simulink model "model2017b"  (R2017b)
settings: Solver=VariableStepAuto  StartTime=0.0  StopTime=10.0  MaxStep=0.001  RelTol=1e-3
values from neighbouring files (symbols this model uses):
  F = 0    [main.m]
  g = 9.81    [main.m]
  l = 1    [main.m]
  M = 0.5    [main.m]
  m = 0.5    [main.m]
  T = 0    [main.m]
settings Model: Creator=mc764  LastModifiedBy=mc764

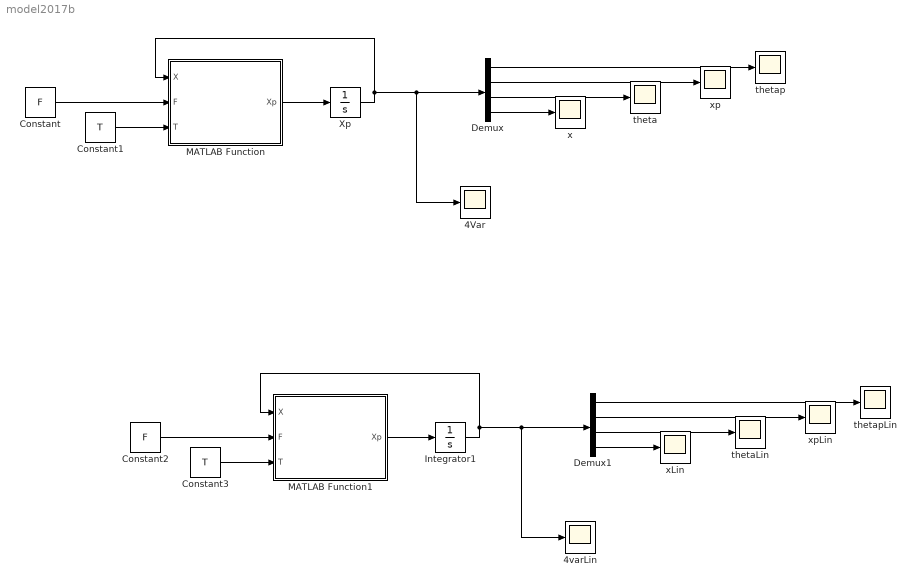
== system model2017b ==
  4Var : Scope
  4varLin : Scope
  Constant : Constant  Value=F
  Constant1 : Constant  Value=T
  Constant2 : Constant  Value=F
  Constant3 : Constant  Value=T
  Demux : Demux
  Demux1 : Demux
  Integrator1 : Integrator  InitialCondition=[0 0 180 0]
  MATLAB Function : MATLAB Function  TreatAsAtomicUnit=on
  MATLAB Function1 : MATLAB Function  TreatAsAtomicUnit=on
  Xp : Integrator  InitialCondition=[0 0 180 0]
  theta : Scope
  thetaLin : Scope
  thetap : Scope
  thetapLin : Scope
  x : Scope
  xLin : Scope
  xp : Scope
  xpLin : Scope
  wires:
  MATLAB Function/1(Xp) -> Xp/1
  Xp/1 -> 4Var/1, Demux/1, MATLAB Function/1(X)
  Constant/1 -> MATLAB Function/2(F)
  Constant1/1 -> MATLAB Function/3(T)
  Demux/1 -> thetap/1
  Demux/2 -> xp/1
  Demux/3 -> theta/1
  Demux/4 -> x/1
  Demux1/4 -> xLin/1
  Constant3/1 -> MATLAB Function1/3(T)
  Integrator1/1 -> 4varLin/1, Demux1/1, MATLAB Function1/1(X)
  Constant2/1 -> MATLAB Function1/2(F)
  Demux1/3 -> thetaLin/1
  Demux1/1 -> thetapLin/1
  Demux1/2 -> xpLin/1
  MATLAB Function1/1(Xp) -> Integrator1/1

== matlab function model2017b/MATLAB Function1 ==
  data: X input; Xp output; F input; T input; m parameter; M parameter; g parameter; l parameter
function Xp  = Segway_Lin0(X, F, T, m, M, g, l)
Xp = zeros([1,4]);
Xp(2) = (m*g*X(3)+F+T/l)/M; % X = (tp xp t x) so Xp = (tpp xpp tp xp)
Xp(1) = ((M+m)*g*l*X(3)+T*(M+m)/m+l*F)/((l^2)*M);
Xp(3) = X(1);
Xp(4) = X(2);
end

== matlab function model2017b/MATLAB Function ==
  data: X input; Xp output; F input; T input; m parameter; M parameter; g parameter; l parameter
function Xp  = Segway_Nolin(X, F, T, m, M, g, l)
Xp = zeros([1,4]);
Xp(2) = (-m*l*(X(1)^2)*sin(X(3))+m*g*cosd(X(3))*sind(X(3))+F+((T*cosd(X(3)))/l))/(M+m-m*(cosd(X(3))^2)); % X = (tp xp t x) so Xp = (tpp xpp tp xp)
Xp(1) = ((M+m)*g*l*sind(X(3))-m*((l*X(1))^2)*cosd(X(3))*sind(X(3))+T*(M+m)/m+l*F*cosd(X(3))/((l^2)*(M+m-m*(cosd(X(3))^2))));
Xp(3) = X(1);
Xp(4) = X(2);
end
